simulink model "exampleSaturationTemperature"  (Simulink 7.6)
settings: Solver=ode45  StartTime=0.0  StopTime=10.0  RelTol=1e-3
libraries: carnot x4
settings Model: Creator=drhf  LastModifiedBy=drhf

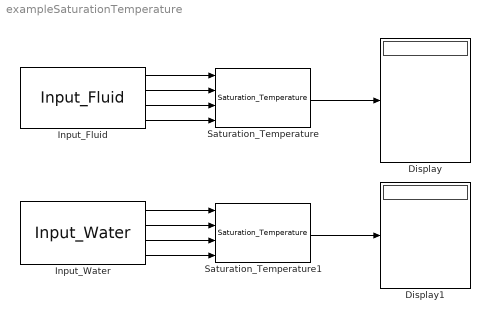
== system exampleSaturationTemperature ==
  Display : Display
  Display1 : Display
  Input_Fluid : carnot/Basic/Material_Properties/Input_Fluid  SystemSampleTime=-1  fluid=air  T=20  p=1e5  x=[0:0.002:0.01]
  Input_Water : carnot/Basic/Material_Properties/Input_Water  SystemSampleTime=-1  T=20  p=1013e2  xd=0
  Saturation_Temperature : carnot/Basic/Material_Properties/Saturation_Temperature  SystemSampleTime=-1
  Saturation_Temperature1 : carnot/Basic/Material_Properties/Saturation_Temperature  SystemSampleTime=-1
  wires:
  Input_Fluid/1 -> Saturation_Temperature/1
  Input_Fluid/2 -> Saturation_Temperature/2
  Input_Fluid/3 -> Saturation_Temperature/3
  Input_Fluid/4 -> Saturation_Temperature/4
  Saturation_Temperature/1 -> Display/1
  Input_Water/1 -> Saturation_Temperature1/1
  Input_Water/2 -> Saturation_Temperature1/2
  Input_Water/3 -> Saturation_Temperature1/3
  Input_Water/4 -> Saturation_Temperature1/4
  Saturation_Temperature1/1 -> Display1/1
